simulink model "different_frequency"  (R2023b)
settings: Solver=VariableStepAuto  StartTime=0.0  StopTime=10.0  RelTol=1e-3
settings Model: Creator=Avijeet Jain  LastModifiedBy=Avijeet Jain

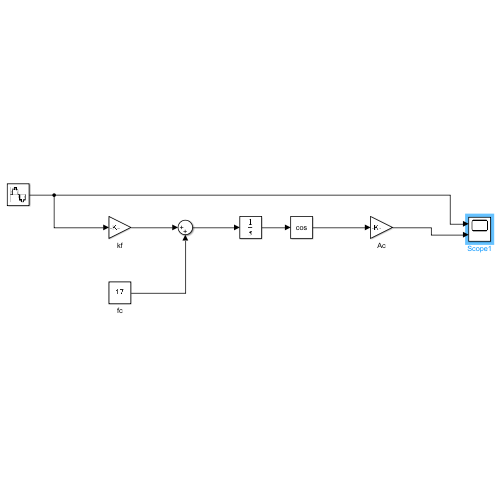
[thumbnail: Simulink's stored preview of the top-level diagram]
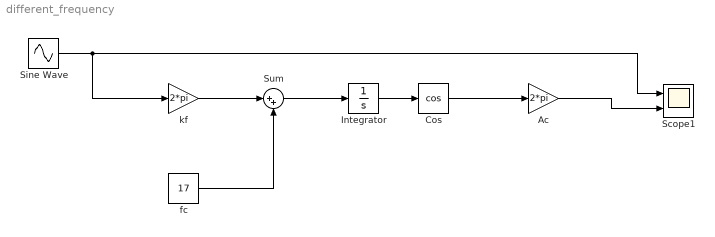
== system different_frequency ==
  Ac : Gain  Gain=2*pi
  Cos : Trigonometry  Operator=cos
  Integrator : Integrator
  Scope1 : Scope  NumInputPorts=2
  Sine Wave : Sin  SampleTime=1/5000
  Sum : Sum  Inputs=|++
  fc : Constant  Value=17
  kf : Gain  Gain=2*pi
  wires:
  Sine Wave/1 -> Scope1/1, kf/1
  kf/1 -> Sum/1
  Sum/1 -> Integrator/1
  Cos/1 -> Ac/1
  Ac/1 -> Scope1/2
  Integrator/1 -> Cos/1
  fc/1 -> Sum/2
